simulink model "I2_05_1_tr_road_sl_avi_R2016a"  (R2016a)
settings: Solver=VariableStepDiscrete  StartTime=0.0  StopTime=Inf  RelTol=1e-3
libraries: visionsinks x3, visiongeotforms x2, dspvision x1
settings Model: Creator=motobe  LastModifiedBy=motobe
settings DataIOCC: LimitDataPoints=on  SaveFormat=Array
settings OptimizationCC: ExpressionDepthLimit=2147483647
settings DebuggingCC: UnderspecifiedInitializationDetection=Classic  MergeDetectMultiDrivingBlocksExec=none  SolverPrmCheckMsg=warning  AllowSymbolicDim=off  StateNameClashWarn=warning
settings HardwareCC: ProdBitPerPointer=32  ProdLargestAtomicFloat=None  ProdIntDivRoundTo=Undefined  ProdEndianess=Unspecified  ProdWordSize=32  ProdHWDeviceType=32-bit Generic
settings ModelReferenceCC: PropagateSignalLabelsOutOfModel=off
settings ConfigComp: CovModelRefEnable=Off  CovSFcnEnable=off

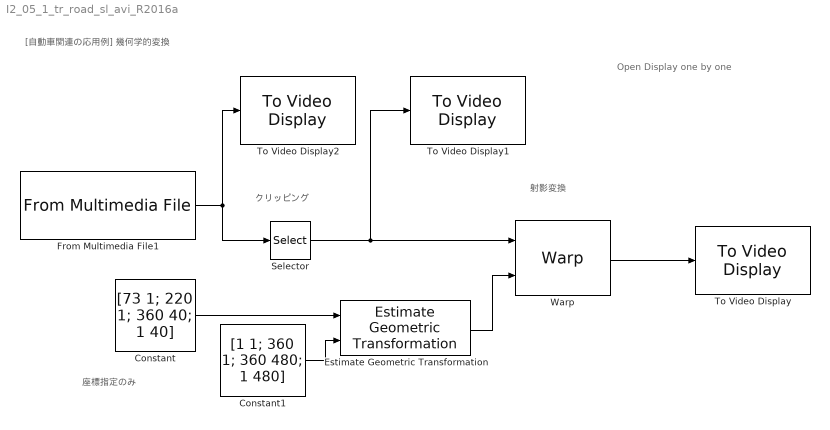
== system I2_05_1_tr_road_sl_avi_R2016a ==
  note: [自動車関連の応用例]
      |     幾何学的変換
  note: Open Display one by one
  note: 座標指定のみ
  note: クリッピング
  note: 射影変換
  Constant : Constant  Value=[73 1; 220 1; 360 40; 1 40]  OutDataTypeStr=single
  Constant1 : Constant  Value=[1 1; 360 1; 360 480; 1 480]  OutDataTypeStr=single
  Estimate Geometric Transformation : visiongeotforms/Estimate Geometric Transformation  tformType=Projective  isRandomSampling=off  algMethod=Random Sample Consensus (RANSAC)  numMethod=Specified value  isStopSampling=off  percentStop=75  distanceAlg=2.5  distanceGeo=2.5  sampleNum=500  maxSampleNum=1000  desiredConfidence=99  isRefineTForm=off  isOutputInlier=off  outDT4IntInput=Obsolete10a  outDT4IntInputActive=Single  isVarSizeAllowed=on  isReleaseMode=on
  From Multimedia File1 : dspvision/From Multimedia File  inputFilename=viplanedeparture.mp4  loop=on  numPlays=inf  outputStreams=Video only  videoDataType=single  audioDataType=int16  inheritSampleTime=off  userDefinedSampleTime=1/30  noAudioOutput=off  isIntensityVideo=off  fourcc=RGB  colorVideoFormat=One multidimensional signal  outputEOF=off  dataOrg=Column-major  audioFrameSize=1024  computeAudioFrameSize=off  outSamplingMode=Frame based
  Selector : Selector  NumberOfDimensions=3  InputPortWidth=3  IndexOptions=Index vector (dialog),Select all,Select all  Indices=[121:160],[140:730],1  OutputSizes=1,1,1
  To Video Display : visionsinks/To Video Display  windowSizeMode=Normal  openAtMdlStart=on  fullScreen=off  videoWindowX=131  videoWindowY=415  saveWindowSize=off  videoWindowWidth=360  videoWindowHeight=349  inputColorFormat=RGB  inputType=Obsolete  imagePorts=One multidimensional signal  OutputDevice=On-screen video monitor  dataOrg=Column-major  isWindowOpen=off
  To Video Display1 : visionsinks/To Video Display  windowSizeMode=Normal  openAtMdlStart=on  fullScreen=off  videoWindowX=52  videoWindowY=435  saveWindowSize=off  videoWindowWidth=360  videoWindowHeight=138  inputColorFormat=RGB  inputType=Obsolete  imagePorts=One multidimensional signal  OutputDevice=On-screen video monitor  dataOrg=Column-major  isWindowOpen=off
  To Video Display2 : visionsinks/To Video Display  windowSizeMode=Normal  openAtMdlStart=on  fullScreen=off  videoWindowX=44  videoWindowY=141  saveWindowSize=off  videoWindowWidth=360  videoWindowHeight=240  inputColorFormat=RGB  inputType=Obsolete  imagePorts=One multidimensional signal  OutputDevice=On-screen video monitor  dataOrg=Column-major  isWindowOpen=off
  Warp : visiongeotforms/Warp  TransformMatrixSource=Input port  TransformMatrix=eye( 3 )  InterpolationMethod=Bilinear  BackgroundFillValue=0  OutputImagePositionSource=Same as input image  OutputImagePosition=[ 1, 1, 512, 512 ]  ROIInputPort=off  ROIValidityOutputPort=off  SimulateUsing=Interpreted execution
  wires:
  From Multimedia File1/1 -> To Video Display2/1, Selector/1
  Warp/1 -> To Video Display/1
  Selector/1 -> Warp/1, To Video Display1/1
  Constant/1 -> Estimate Geometric Transformation/1
  Constant1/1 -> Estimate Geometric Transformation/2
  Estimate Geometric Transformation/1 -> Warp/2
